simulink model "PILcontroller_block"  (R2019b)
settings: Solver=FixedStepAuto  StartTime=0.0  StopTime=30  RelTol=1e-3  EnableMultiTasking=on
undefined symbols (not defined in the file): Discovery, Serial, STM32F4
libraries: pil_lib x1
settings Model: Creator=alelu  LastModifiedBy=alelu
settings SolverCC: ZeroCrossAlgorithm=Adaptive  AutoInsertRateTranBlk=on  InsertRTBMode=Never (minimum delay)
settings OptimizationCC: EnhancedBackFolding=on  PassReuseOutputArgsAs=Individual arguments  ZeroExternalMemoryAtStartup=off  ZeroInternalMemoryAtStartup=off  MaxStackSize=64  OptimizeBlockOrder=speed  DifferentSizesBufferReuse=on  OptimizationCustomize=off  EfficientTunableParamExpr=on
settings DebuggingCC: ArtificialAlgebraicLoopMsg=none  ParameterTunabilityLossMsg=error  ModelReferenceExtraNoncontSigs=none
settings HardwareCC: ProdBitPerPointer=32  ProdBitPerSizeT=32  ProdBitPerPtrDiffT=32  ProdLargestAtomicInteger=Long  ProdLargestAtomicFloat=Double  ProdWordSize=32  ProdHWDeviceType=ARM Compatible->ARM Cortex
settings ModelReferenceCC: ModelReferenceMinAlgLoopOccurrences=on  PropagateSignalLabelsOutOfModel=off
settings SFSimCC: MATLABDynamicMemAlloc=off  CustomCodeUndefinedFunction=UseInterfaceOnly
settings RTWCC: SystemTargetFile=ert.tlc  HardwareBoard=STM32F4-Discovery  TLCOptions=-aInlineSetEventsForThisBaseRateFcn=TLC_FALSE -aSuppressMultiTaskScheduler=TLC_FALSE -aRateBasedStepFcn=1  TemplateMakefile=ert_default_tmf  GenerateReport=on  Toolchain=GNU Tools for ARM Embedded Processors  IncludeHyperlinkInReport=on  LaunchReport=on  CreateSILPILBlock=PIL  GenerateTraceInfo=on  GenerateTraceReport=on  GenerateTraceReportSl=on  GenerateTraceReportSf=on  GenerateTraceReportEml=on
settings CodeAppCC: ForceParamTrailComments=on  IgnoreCustomStorageClasses=off  OperatorAnnotations=on  SimulinkDataObjDesc=on  SFDataObjDesc=on  InsertBlockDesc=on
settings ERTTargetCC: CodeReplacementLibrary=ARM Cortex-M (Optimized)

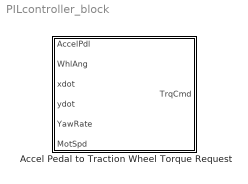
== system PILcontroller_block ==
  Accel Pedal to Traction Wheel Torque Request : Subsystem  DialogController=pil_create_dialog  LoadFcn=|
      | try
      |    if ~strcmp(rtw.pil.getPILVersion, '9.7 (R2019b)_13')
      |       set_param(gcb, 'DialogController', '');
      |       set_param(gcb, 'DialogControllerArgs', '');
      |    end
      | catch e
      |       set_param(gcb, 'DialogController', '');
      |       set_param(gcb, 'DialogControllerArgs', '');
      | end
      mask help: PIL:pil:XILBlockMaskDesc
      mask Display: disp('PIL');

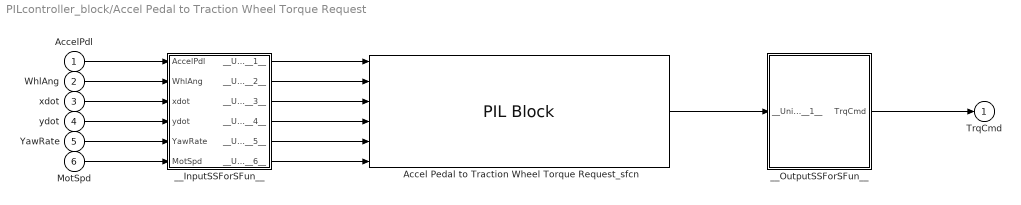
== system PILcontroller_block/Accel Pedal to Traction Wheel Torque Request ==
  AccelPdl : Inport
  WhlAng : Inport  Port=2
  xdot : Inport  Port=3
  ydot : Inport  Port=4
  YawRate : Inport  Port=5
  MotSpd : Inport  Port=6
  Accel Pedal to Traction Wheel Torque Request_sfcn : pil_lib/PIL Block  SimulationMode=PIL  IsTopModelPIL=off  CodeDir=C:\Users\Alessandro\Documents\GitHub\electronic-differential\integrated_system\Accel_ert_rtw  AnchorDir=C:\Users\Alessandro\Documents\GitHub\electronic-differential\integrated_system  ConfigName=STM32F4-Discovery (Serial)  XrelIsTopModelCode=on  XrelIsReusable=off  XrelDWorkNames={}  XrelDWorkTypes={}  XrelModelArgVals={}  XrelOrderedParamNames={}
      settings: SourceProductName=Simulink Coder  SourceProductBaseCode=RT
  __InputSSForSFun__ : Subsystem
  __OutputSSForSFun__ : Subsystem
  TrqCmd : Outport  VectorParamsAs1DForOutWhenUnconnected=off
  wires:
  AccelPdl/1 -> __InputSSForSFun__/1(AccelPdl)
  WhlAng/1 -> __InputSSForSFun__/2(WhlAng)
  xdot/1 -> __InputSSForSFun__/3(xdot)
  ydot/1 -> __InputSSForSFun__/4(ydot)
  YawRate/1 -> __InputSSForSFun__/5(YawRate)
  MotSpd/1 -> __InputSSForSFun__/6(MotSpd)
  __InputSSForSFun__/1(__UniqueOutportName__1__) -> Accel Pedal to Traction Wheel Torque Request_sfcn/1
  __InputSSForSFun__/2(__UniqueOutportName__2__) -> Accel Pedal to Traction Wheel Torque Request_sfcn/2
  __InputSSForSFun__/3(__UniqueOutportName__3__) -> Accel Pedal to Traction Wheel Torque Request_sfcn/3
  __InputSSForSFun__/4(__UniqueOutportName__4__) -> Accel Pedal to Traction Wheel Torque Request_sfcn/4
  __InputSSForSFun__/5(__UniqueOutportName__5__) -> Accel Pedal to Traction Wheel Torque Request_sfcn/5
  __InputSSForSFun__/6(__UniqueOutportName__6__) -> Accel Pedal to Traction Wheel Torque Request_sfcn/6
  Accel Pedal to Traction Wheel Torque Request_sfcn/1 -> __OutputSSForSFun__/1(__UniqueInportName__1__)
  __OutputSSForSFun__/1(TrqCmd) -> TrqCmd/1

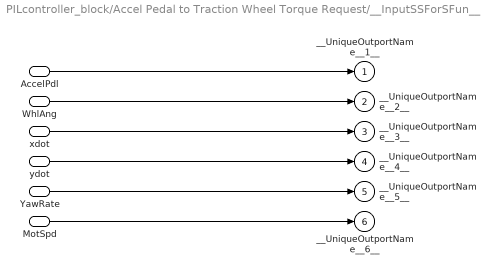
== system PILcontroller_block/Accel Pedal to Traction Wheel Torque Request/__InputSSForSFun__ ==
  AccelPdl : Inport
  WhlAng : Inport  Port=2
  xdot : Inport  Port=3
  ydot : Inport  Port=4
  YawRate : Inport  Port=5
  MotSpd : Inport  Port=6
  __UniqueOutportName__1__ : Outport
  __UniqueOutportName__2__ : Outport  Port=2
  __UniqueOutportName__3__ : Outport  Port=3
  __UniqueOutportName__4__ : Outport  Port=4
  __UniqueOutportName__5__ : Outport  Port=5
  __UniqueOutportName__6__ : Outport  Port=6
  wires:
  AccelPdl/1 -> __UniqueOutportName__1__/1
  WhlAng/1 -> __UniqueOutportName__2__/1
  xdot/1 -> __UniqueOutportName__3__/1
  ydot/1 -> __UniqueOutportName__4__/1
  YawRate/1 -> __UniqueOutportName__5__/1
  MotSpd/1 -> __UniqueOutportName__6__/1

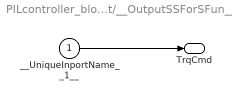
== system PILcontroller_block/Accel Pedal to Traction Wheel Torque Request/__OutputSSForSFun__ ==
  __UniqueInportName__1__ : Inport
  TrqCmd : Outport  VectorParamsAs1DForOutWhenUnconnected=off
  wires:
  __UniqueInportName__1__/1 -> TrqCmd/1
